simulink model "Steven"  (R2022a)
settings: Solver=VariableStepAuto  StartTime=0.0  StopTime=20  RelTol=1e-3
values from neighbouring files (symbols this model uses):
  A = [-1.9311E-02    8.8157   -3.217E+01   -5.7499E-01 ... (first row only)    [Steven_PreLoadFcn.m]
  B = [ 1.737E-01   0.1 ... (first row only)    [Steven_PreLoadFcn.m]
  C = [0   1  0   0 ... (first row only)    [Steven_PreLoadFcn.m]
  D = zeros(4,2)    [Steven_PreLoadFcn.m]
  I_C = eye(4)    [Steven_PreLoadFcn.m]
undefined symbols (not defined in the file or in its folder): sysID_DAQ
libraries: slpidlib x2
settings Model: Creator=user  LastModifiedBy=user
settings DataIOCC: ReturnWorkspaceOutputs=off

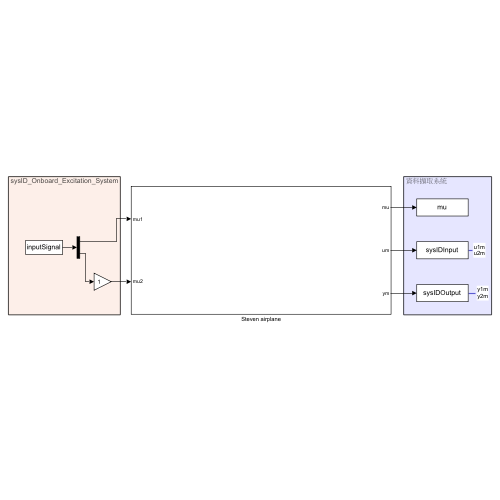
[thumbnail: Simulink's stored preview of the top-level diagram]
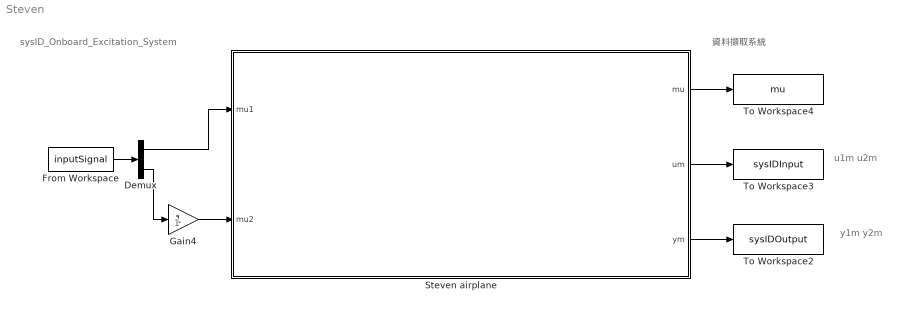
== system Steven ==
  note: sysID_Onboard_Excitation_System
  note: 資料擷取系統
  note: u1m
      | u2m
  note: 1
  note: y1m
      | y2m
  Demux : Demux  Outputs=2
  From Workspace : FromWorkspace  VariableName=inputSignal  OutputAfterFinalValue=Holding final value
  Gain4 : Gain
  Steven airplane : Subsystem
  To Workspace2 : ToWorkspace  VariableName=sysIDOutput  SaveFormat=Timeseries  SampleTime=sysID_DAQ.sampleTime
  To Workspace3 : ToWorkspace  VariableName=sysIDInput  SaveFormat=Timeseries  SampleTime=sysID_DAQ.sampleTime
  To Workspace4 : ToWorkspace  VariableName=mu  SaveFormat=Timeseries  SampleTime=sysID_DAQ.sampleTime
  wires:
  Steven airplane/1(mu) -> To Workspace4/1
  Demux/1 -> Steven airplane/1(mu1)
  Gain4/1 -> Steven airplane/2(mu2)
  Demux/2 -> Gain4/1
  Steven airplane/3(ym) -> To Workspace2/1
  Steven airplane/2(um) -> To Workspace3/1
  From Workspace/1 -> Demux/1

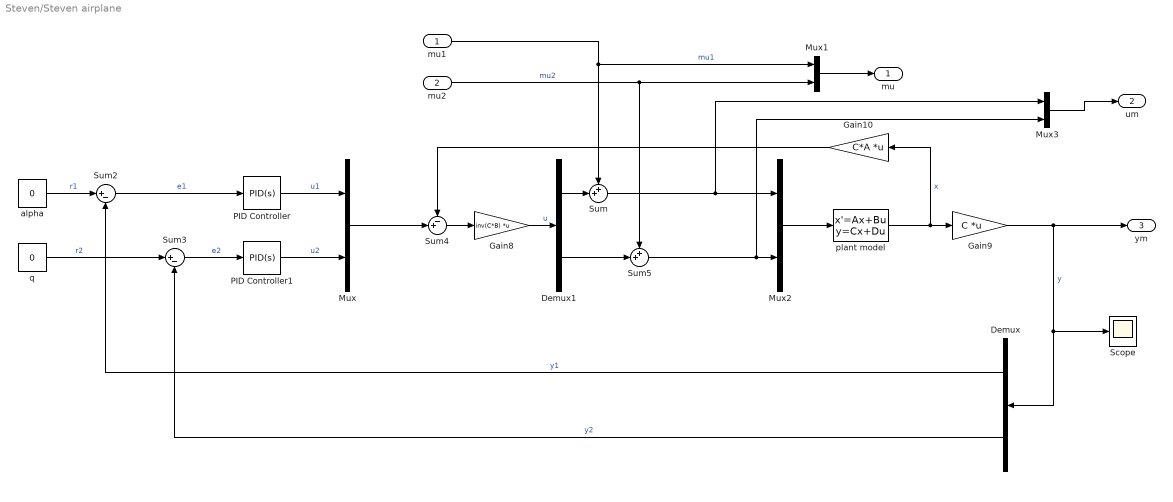
== system Steven/Steven airplane ==
  mu1 : Inport
  mu2 : Inport  Port=2
  Demux : Demux  Outputs=2
  Demux1 : Demux  Outputs=2
  Gain10 : Gain  Gain=C*A  Multiplication=Matrix(K*u) (u vector)
  Gain8 : Gain  Gain=inv(C*B)  Multiplication=Matrix(K*u) (u vector)
  Gain9 : Gain  Gain=C  Multiplication=Matrix(K*u) (u vector)
  Mux{,1..3} (4 alike) : Mux  Inputs=2
  PID Controller : slpidlib/PID Controller  Controller=PID  Form=Parallel  TimeDomain=Continuous-time  UseExternalTs=off  SampleTime=-1  IntegratorMethod=Forward Euler  FilterMethod=Forward Euler  ControllerParametersSource=internal  P=2.64151778914193  I=0.058111644364251  UseKiTs=off  D=-0.107160889147502  N=2.51188643150958  UseFilter=on  TunerSelectOption=Transfer Function Based (PID Tuner App)  InitialConditionSource=internal  InitialConditionForIntegrator=0  InitialConditionForFilter=0  DifferentiatorICPrevScaledInput=0  ExternalReset=none  TrackingMode=off  Kt=1  LimitOutput=off  SatLimitsSource=internal  UpperSaturationLimit=inf  LowerSaturationLimit=-inf  LinearizeAsGain=on  AntiWindupMode=none  Kb=1  POutMin=[]  POutMax=[]  IOutMin=[]  IOutMax=[]  DOutMin=[]  DOutMax=[]  NOutMin=[]  NOutMax=[]  SumOutMin=[]  SumOutMax=[]  SaturationOutMin=[]  SaturationOutMax=[]  PParamMin=[]  PParamMax=[]  IParamMin=[]  IParamMax=[]  DParamMin=[]  DParamMax=[]  NParamMin=[]  NParamMax=[]  KbParamMin=[]  KbParamMax=[]  KtParamMin=[]  KtParamMax=[]  KbOutMin=[]  KbOutMax=[]  KtOutMin=[]  KtOutMax=[]  IntegratorOutMin=[]  IntegratorOutMax=[]  FilterOutMin=[]  FilterOutMax=[]  SumI1OutMin=[]  SumI1OutMax=[]  SumI2OutMin=[]  SumI2OutMax=[]  SumI3OutMin=[]  SumI3OutMax=[]  SumI4OutMin=[]  SumI4OutMax=[]  SumDOutMin=[]  SumDOutMax=[]  DifferentiatorOutMin=[]  DifferentiatorOutMax=[]  FilterDiffOutCoefMin=[]  FilterDiffOutCoefMax=[]  ReciprocalOutMin=[]  ReciprocalOutMax=[]  SumDenOutMin=[]  SumDenOutMax=[]  SumNumOutMin=[]  SumNumOutMax=[]  DivideOutMin=[]  DivideOutMax=[]  UdiffTsProdOutMin=[]  UdiffTsProdOutMax=[]  NTsProdOutMin=[]  NTsProdOutMax=[]  UintegralTsProdOutMin=[]  UintegralTsProdOutMax=[]  UngainTsProdOutMin=[]  UngainTsProdOutMax=[]  IntegratorContinuousStateAttributes=''  IntegratorStateMustResolveToSignalObject=off  IntegratorRTWStateStorageClass=Auto  FilterContinuousStateAttributes=''  FilterStateMustResolveToSignalObject=off  FilterRTWStateStorageClass=Auto  ParallelPVariant=InternalParameters  IdealPVariant=Disabled  IVariant=InternalParameters  DVariant=InternalParameters  IntegratorVariant=Continuous  SatVariant=Disabled  AWVariant=Passthrough  PCopyVariant=Disabled  TRVariant=Disabled  FdbkBlocksVariant=Forward  IdealPFdbkVariant=Disabled  SatFdbkVariant=Disabled  DerivativeFilterVariant=ContFilter  NVariant=InternalParameters  NCopyVariant=Disabled  FilterICVariant=InternalICsFilter  IntegratorICVariant=InternalICs  ExternalResetVariant=Disabled  TRSumVariant=Passthrough  SumFdbkVariant=Disabled  SumVariant=Sum_PID  TsampFilterVariant=InternalTs  TsampNgainVariant=Passthrough  TsampIntegralVariant=Passthrough  ExternalSaturationOutDataTypeStr=Inherit: Same as second input  aMode=0
  PID Controller1 : slpidlib/PID Controller  Controller=PID  Form=Parallel  TimeDomain=Continuous-time  UseExternalTs=off  SampleTime=-1  IntegratorMethod=Forward Euler  FilterMethod=Forward Euler  ControllerParametersSource=internal  P=9.53803500565493  I=16.8470505938331  UseKiTs=off  D=0.181138103439247  N=36.46824066771  UseFilter=on  TunerSelectOption=Transfer Function Based (PID Tuner App)  InitialConditionSource=internal  InitialConditionForIntegrator=0  InitialConditionForFilter=0  DifferentiatorICPrevScaledInput=0  ExternalReset=none  TrackingMode=off  Kt=1  LimitOutput=off  SatLimitsSource=internal  UpperSaturationLimit=inf  LowerSaturationLimit=-inf  LinearizeAsGain=on  AntiWindupMode=none  Kb=1  POutMin=[]  POutMax=[]  IOutMin=[]  IOutMax=[]  DOutMin=[]  DOutMax=[]  NOutMin=[]  NOutMax=[]  SumOutMin=[]  SumOutMax=[]  SaturationOutMin=[]  SaturationOutMax=[]  PParamMin=[]  PParamMax=[]  IParamMin=[]  IParamMax=[]  DParamMin=[]  DParamMax=[]  NParamMin=[]  NParamMax=[]  KbParamMin=[]  KbParamMax=[]  KtParamMin=[]  KtParamMax=[]  KbOutMin=[]  KbOutMax=[]  KtOutMin=[]  KtOutMax=[]  IntegratorOutMin=[]  IntegratorOutMax=[]  FilterOutMin=[]  FilterOutMax=[]  SumI1OutMin=[]  SumI1OutMax=[]  SumI2OutMin=[]  SumI2OutMax=[]  SumI3OutMin=[]  SumI3OutMax=[]  SumI4OutMin=[]  SumI4OutMax=[]  SumDOutMin=[]  SumDOutMax=[]  DifferentiatorOutMin=[]  DifferentiatorOutMax=[]  FilterDiffOutCoefMin=[]  FilterDiffOutCoefMax=[]  ReciprocalOutMin=[]  ReciprocalOutMax=[]  SumDenOutMin=[]  SumDenOutMax=[]  SumNumOutMin=[]  SumNumOutMax=[]  DivideOutMin=[]  DivideOutMax=[]  UdiffTsProdOutMin=[]  UdiffTsProdOutMax=[]  NTsProdOutMin=[]  NTsProdOutMax=[]  UintegralTsProdOutMin=[]  UintegralTsProdOutMax=[]  UngainTsProdOutMin=[]  UngainTsProdOutMax=[]  IntegratorContinuousStateAttributes=''  IntegratorStateMustResolveToSignalObject=off  IntegratorRTWStateStorageClass=Auto  FilterContinuousStateAttributes=''  FilterStateMustResolveToSignalObject=off  FilterRTWStateStorageClass=Auto  ParallelPVariant=InternalParameters  IdealPVariant=Disabled  IVariant=InternalParameters  DVariant=InternalParameters  IntegratorVariant=Continuous  SatVariant=Disabled  AWVariant=Passthrough  PCopyVariant=Disabled  TRVariant=Disabled  FdbkBlocksVariant=Forward  IdealPFdbkVariant=Disabled  SatFdbkVariant=Disabled  DerivativeFilterVariant=ContFilter  NVariant=InternalParameters  NCopyVariant=Disabled  FilterICVariant=InternalICsFilter  IntegratorICVariant=InternalICs  ExternalResetVariant=Disabled  TRSumVariant=Passthrough  SumFdbkVariant=Disabled  SumVariant=Sum_PID  TsampFilterVariant=InternalTs  TsampNgainVariant=Passthrough  TsampIntegralVariant=Passthrough  ExternalSaturationOutDataTypeStr=Inherit: Same as second input  aMode=0
  Scope : Scope
  Sum : Sum  Inputs=++|
  Sum2 : Sum  Inputs=|+-
  Sum3 : Sum  Inputs=|+-
  Sum4 : Sum  Inputs=-+|
  Sum5 : Sum  Inputs=++|
  alpha : Constant  Value=0
  plant model : StateSpace  A=A  B=B  C=I_C  D=D  InitialCondition=0
  q : Constant  Value=0
  mu : Outport
  um : Outport  Port=2
  ym : Outport  Port=3
  wires:
  mu2/1 -> Sum5/1, Mux1/2  "mu2"
  mu1/1 -> Sum/1, Mux1/1  "mu1"
  Gain9/1 -> ym/1, Scope/1, Demux/1  "y"
  Mux1/1 -> mu/1
  plant model/1 -> Gain10/1, Gain9/1  "x"
  Mux/1 -> Sum4/2
  Sum4/1 -> Gain8/1
  Gain10/1 -> Sum4/1
  PID Controller/1 -> Mux/1  "u1"
  alpha/1 -> Sum2/1  "r1"
  Sum2/1 -> PID Controller/1  "e1"
  Demux/1 -> Sum2/2  "y1"
  q/1 -> Sum3/1  "r2"
  Sum3/1 -> PID Controller1/1  "e2"
  Demux/2 -> Sum3/2  "y2"
  Mux2/1 -> plant model/1
  PID Controller1/1 -> Mux/2  "u2"
  Gain8/1 -> Demux1/1  "u"
  Demux1/2 -> Sum5/2
  Sum/1 -> Mux3/1, Mux2/1
  Sum5/1 -> Mux3/2, Mux2/2
  Demux1/1 -> Sum/2
  Mux3/1 -> um/1
